simulink model "OpAmp_Inverted_Amplifier_741"  (R2020a)
settings: Solver=VariableStepAuto  StartTime=0.0  StopTime=10  RelTol=1e-3
libraries: fl_lib x5, ee_lib x3, nesl_utility x3, slctrlblks x1
settings Model: Creator=ashwin  LastModifiedBy=ashwin

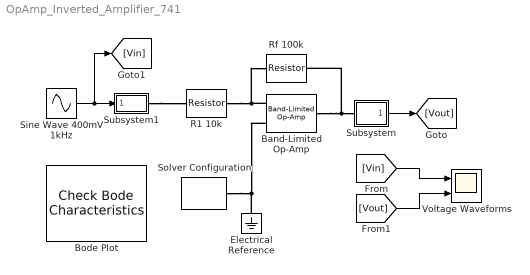
== system OpAmp_Inverted_Amplifier_741 ==
  Band-Limited Op-Amp : ee_lib/Integrated Circuits/Band-Limited Op-Amp  A=50000  Rin=0.3 MOhm  Rout=100 Ohm  Vmin=-15 V  Vmax=15 V  Vdotmax=0.2e6 V/s  f=250 kHz  V0=0 V
      settings: SourceProductBaseCode=PS
  Bode Plot : slctrlblks/Model Verification/Check Bode  Characteristics  InstantiateOnLoad=on  SaveOperatingPoints=off  LinearizationIOs={'/Sine Wave 400mV 1kHz', 1, 'in', 'off', '';'/Subsystem', 1, 'out', 'off', ''}  LinearizeAt=SnapshotTimes  SnapshotTimes=[5]  TriggerType=rising  SampleTime=auto  RateConversionMethod=zoh  PreWarpFreq=10  UseExactDelayModel=off  UseFullBlockNameLabels=off  UseBusSignalLabels=off  enabled=on  stopWhenAssertionFail=off  export=off  ViewDlgPos=[100 200 510 390]  OpenViewOnLoad=off  LaunchViewOnOpen=off  FrequencyUnits=rad/s  MagnitudeUnits=dB  PhaseUnits=deg  TimeUnits=seconds  EnableUpperBound=off  UpperBoundFrequencies=[]  UpperBoundMagnitudes=[]  EnableLowerBound=off  LowerBoundFrequencies=[]  LowerBoundMagnitudes=[]
  Electrical Reference : fl_lib/Electrical/Electrical Elements/Electrical Reference
  R1 10k : ee_lib/Passive/Resistor  R=10 kOhm  R_tol=5  enable_R_tol=0  tol_distribution=1  nSigma=4  enable_operating_limits=0  operating_limit_action=2  max_working_voltage=100 V  power_rating=1 W  enable_faults=0  fault_action=1  R_faulted=inf Ohm  enable_temporal_fault=0  t_fault=1 s  enable_behavioral_fault=0  max_permissible_current=1 A  t_fail_on_current=1 s  noise_mode=0  sample_time=1e-3 s  repeatability=1  auto_seed=3099927149  user_seed=0  Tdevice=25 degC  alpha=3.93e-3 1/K  Tmeas=25 degC  thermal_mass=100 J/K  power_derating_T1=70 degC  power_derating_T2=155 degC  operating_temperature_range_vec=[-50, 150] degC  temperature_specify=off  temperature_priority=High  temperature=298.15 K  temperature_nominal_specify=off  temperature_nominal_unit=K  temperature_nominal_value=1
  Rf 100k : ee_lib/Passive/Resistor  R=100 kOhm  R_tol=5  enable_R_tol=0  tol_distribution=1  nSigma=4  enable_operating_limits=0  operating_limit_action=2  max_working_voltage=100 V  power_rating=1 W  enable_faults=0  fault_action=1  R_faulted=inf Ohm  enable_temporal_fault=0  t_fault=1 s  enable_behavioral_fault=0  max_permissible_current=1 A  t_fail_on_current=1 s  noise_mode=0  sample_time=1e-3 s  repeatability=1  auto_seed=2033606855  user_seed=0  Tdevice=25 degC  alpha=3.93e-3 1/K  Tmeas=25 degC  thermal_mass=100 J/K  power_derating_T1=70 degC  power_derating_T2=155 degC  operating_temperature_range_vec=[-50, 150] degC  temperature_specify=off  temperature_priority=High  temperature=298.15 K  temperature_nominal_specify=off  temperature_nominal_unit=K  temperature_nominal_value=1
  Sine Wave 400mV 1kHz : Sin  Amplitude=0.2  Frequency=2*pi*100  SampleTime=0
  Solver Configuration : nesl_utility/Solver Configuration  PhysicalDomain=network_engine_domain  SubClassName=solver  LeftPortType=input  RightPortType=generic  Tones=[]  Harmonics=[]  SimulateNoise=off  Profile=off  UseLocalSampling=off  EnableSwitchedLinearOptims=on  FrequencyDomain=off  UseCCode=off  RelTol=0.001  AbsTol=1e-06  MinStep=1e-09  ToWorkspace=off  RevertToSquareIcSolve=off  NumHomotopyIterations=100  PhasorMode=off  PhasorModeNumHarmonics=1  DoDC=off  ResidualTolerance=1e-09  UseLocalSolver=off  LocalSolverChoice=NE_BACKWARD_EULER_ADVANCER  LocalSolverSampleTime=0.001  DoFixedCost=off  MaxNonlinIter=3  MaxModeIter=2  LinearAlgebra=auto  EquationFormulation=NE_TIME_EF  DelaysMemoryBudget=1024  AutomaticFiltering=on  FilteringTimeConstant=0.001  PartitionStorageMethod=AS_NEEDED  PartitionMemoryBudget=1024  PartitionMethod=ROBUST
  Subsystem : Subsystem
      mask Display: disp('Vout');
  Subsystem1 : Subsystem
      mask Display: disp('Vin');
  Voltage Waveforms : Scope  NumInputPorts=2
  wires:
  Sine Wave 400mV 1kHz/1 -> [Vin], Subsystem1/1(input0)
  Subsystem/1(output) -> [Vout]
  [Vin] -> Voltage Waveforms/1
  [Vout] -> Voltage Waveforms/2
  connections:
  R1 10k/RConn1 -- Band-Limited Op-Amp/LConn2 -- Rf 100k/LConn1
  Electrical Reference/LConn1 -- Band-Limited Op-Amp/LConn1 -- Solver Configuration/RConn1
  Subsystem/LConn1 -- Band-Limited Op-Amp/RConn1 -- Rf 100k/RConn1
  Subsystem1/RConn1 -- R1 10k/LConn1

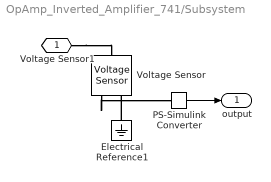
== system OpAmp_Inverted_Amplifier_741/Subsystem ==
  Electrical Reference1 : fl_lib/Electrical/Electrical Elements/Electrical Reference
  PS-Simulink Converter : nesl_utility/PS-Simulink Converter  PhysicalDomain=network_engine_domain  SubClassName=ps_output  LeftPortType=input  RightPortType=output  PseudoPeriodic=off  Frequencies=[]  Unit=inherit  AffineConversion=off
  Voltage Sensor : fl_lib/Electrical/Electrical Sensors/Voltage Sensor
  Voltage Sensor1 : PMIOPort  Side=Left
  output : Outport
  wires:
  PS-Simulink Converter/1 -> output/1
  connections:
  Voltage Sensor1/RConn1 -- Voltage Sensor/LConn1
  Voltage Sensor/RConn1 -- PS-Simulink Converter/LConn1
  Electrical Reference1/LConn1 -- Voltage Sensor/RConn2

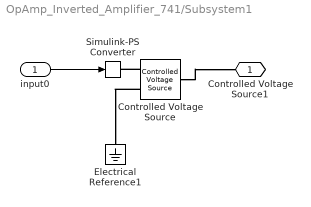
== system OpAmp_Inverted_Amplifier_741/Subsystem1 ==
  input0 : Inport
  Controlled Voltage Source : fl_lib/Electrical/Electrical Sources/Controlled Voltage Source
  Electrical Reference1 : fl_lib/Electrical/Electrical Elements/Electrical Reference
  Simulink-PS Converter : nesl_utility/Simulink-PS Converter  PhysicalDomain=network_engine_domain  SubClassName=ps_input  LeftPortType=input  RightPortType=output  PseudoPeriodic=off  Frequencies=[]  NoiseDistribution=none  NoiseParameters=[]  Unit=1  AffineConversion=off  FilteringAndDerivatives=provide  SimscapeFilterOrder=1  InputFilterTimeConstant=0.001  UdotUserProvided=0
  Controlled Voltage Source1 : PMIOPort  Side=Right
  wires:
  input0/1 -> Simulink-PS Converter/1
  connections:
  Controlled Voltage Source/RConn2 -- Electrical Reference1/LConn1
  Controlled Voltage Source/LConn1 -- Controlled Voltage Source1/RConn1
  Controlled Voltage Source/RConn1 -- Simulink-PS Converter/RConn1
